simulink model "controled_robot"  (R2018a)
settings: Solver=FixedStepAuto  StartTime=0.0  StopTime=20  FixedStep=0.0001  MaxStep=5e-3  RelTol=1e-3
undefined symbols (not defined in the file or in its folder): DiscIntNeverNeededParam, Forward_Dynamics
libraries: simulink x2
settings Model: Creator=julien  LastModifiedBy=quentin
settings SolverCC: AutoInsertRateTranBlk=on
settings DataIOCC: ReturnWorkspaceOutputs=on  ReturnWorkspaceOutputsName=tpe1c572a4_15fe_4767_8dc5_e730d6ee611a  LoggingIntervals=[10, 20]
settings CodeAppCC: StateflowObjectComments=on

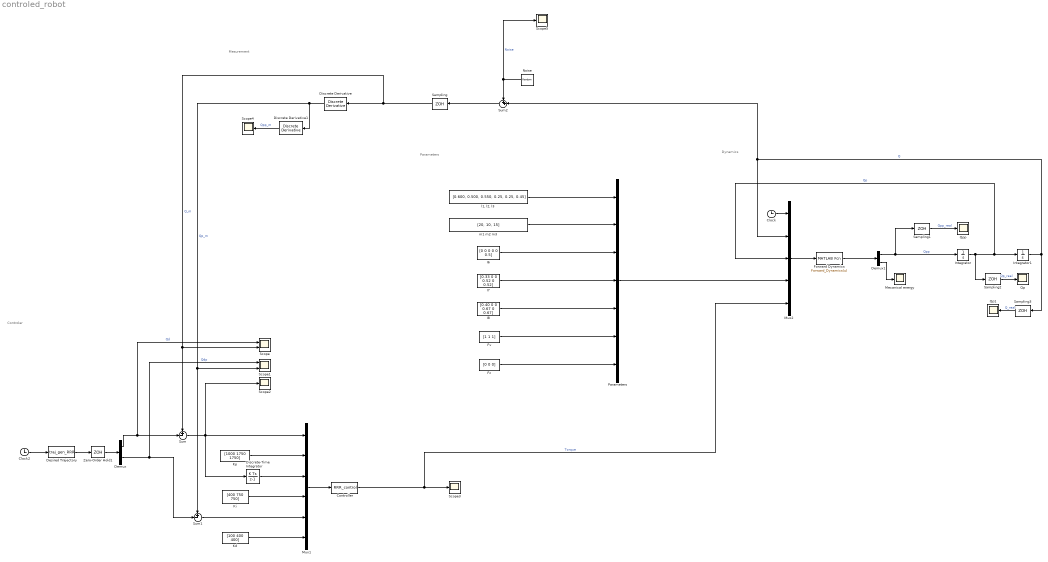
== system controled_robot ==
  note: Parameters
  note: Dynamics
  note: Controler
  note: Mesurement
  Clock : Clock
  Clock2 : Clock
  "Controller " : MATLABFcn  MATLABFcn=RRR_control
  Demux : Demux  Outputs=[3 3]
  Demux1 : Demux  Outputs=[3, 3]
  Desired Trajectory : MATLABFcn  MATLABFcn=traj_gen_RRR  OutputDimensions=6
  Discrete Derivative : simulink/Discrete/Discrete Derivative  gainval=1  ICPrevScaledInput=0.0  OutMin=[]  OutMax=[]  OutDataType=fixdt(1, 16)  OutScaling=2^-10  DoSatur=off
  Discrete Derivative1 : simulink/Discrete/Discrete Derivative  gainval=1  ICPrevScaledInput=0.0  OutMin=[]  OutMax=[]  OutDataType=fixdt(1, 16)  OutScaling=2^-10  DoSatur=off
  Discrete-Time Integrator : DiscreteIntegrator  SampleTime=0.001  ICPrevOutput=DiscIntNeverNeededParam  ICPrevScaledInput=DiscIntNeverNeededParam
  Fc : Constant  Value=[0 0 0]
  Forward Dynamics : MATLABFcn  MATLABFcn=Forward_Dynamics(u)  OutputDimensions=6
  Fv : Constant  Value=[1 1 1]
  I6 : Constant  Value=[0 0 0 0 0 0.5]
  I7 : Constant  Value=[0.33 0 0 0.52 0 0.52]
  I8 : Constant  Value=[0.40 0 0 0.67 0 0.67]
  Integrator : Integrator  InitialCondition=[0,0,0]
  Integrator1 : Integrator  InitialCondition=[0, pi/2, 0.1]
  Kd : Constant  Value=[100 400 400]
  Ki : Constant  Value=[400 750 750]
  Kp : Constant  Value=[1000 1750 1750]
  Mecanical energy : Scope
  Mux1 : Mux  Inputs=6
  Mux2 : Mux  Inputs=5
  Noise : RandomNumber  Mean=[0 0 0]  Variance=1e-3*pi/180*1e-3*pi/180 * [1 1 1]  Seed=[1 2 3]  SampleTime=0.001  VectorParams1D=off
  Parameters : Mux  Inputs=7
  Qp : Scope
  Qp1 : Scope
  Qpp : Scope
  Sampling{,1..3} (4 alike) : ZeroOrderHold  SampleTime=0.001
  Scope : Scope  NumInputPorts=2
  Scope1 : Scope  NumInputPorts=2
  Scope{2..5} (4 alike) : Scope
  Sum : Sum  Inputs=+-|
  Sum1 : Sum  Inputs=+-|
  Sum2 : Sum  Inputs=++|
  Zero-Order Hold1 : ZeroOrderHold  SampleTime=0.001
  "l1, l2, l3" : Constant  Value=[0.600, 0.500, 0.550, 0.25, 0.25, 0.45]
  m1 m2 m3 : Constant  Value=[20, 10, 15]
  wires:
  Clock/1 -> Mux2/1
  Mux2/1 -> Forward Dynamics/1
  Integrator/1 -> Sampling2/1, Mux2/3, Integrator1/1  "Qp"
  Integrator1/1 -> Sampling3/1, Sum2/2, Mux2/2  "Q"
  Clock2/1 -> Desired Trajectory/1
  Desired Trajectory/1 -> Zero-Order Hold1/1
  Demux/1 -> Scope/1, Sum/2  "Qd"
  Demux/2 -> Scope1/1, Sum1/2  "Qdp"
  Sum/1 -> Discrete-Time Integrator/1, Scope2/1, Mux1/1
  Mux1/1 -> "Controller "/1
  Discrete-Time Integrator/1 -> Mux1/3
  Sum1/1 -> Mux1/5
  Kp/1 -> Mux1/2
  Ki/1 -> Mux1/4
  Kd/1 -> Mux1/6
  Forward Dynamics/1 -> Demux1/1
  Demux1/1 -> Sampling1/1, Integrator/1  "Qpp"
  Demux1/2 -> Mecanical energy/1
  "l1, l2, l3"/1 -> Parameters/1
  m1 m2 m3/1 -> Parameters/2
  I6/1 -> Parameters/3
  I7/1 -> Parameters/4
  I8/1 -> Parameters/5
  Fv/1 -> Parameters/6
  Fc/1 -> Parameters/7
  "Controller "/1 -> Scope3/1, Mux2/5  "Torque"
  Parameters/1 -> Mux2/4
  Sampling/1 -> Scope/2, Sum/1, Discrete Derivative/1  "Q_m"
  Discrete Derivative/1 -> Discrete Derivative1/1, Sum1/1, Scope1/2  "Qp_m"
  Zero-Order Hold1/1 -> Demux/1
  Sum2/1 -> Sampling/1
  Noise/1 -> Scope5/1, Sum2/1  "Noise"
  Discrete Derivative1/1 -> Scope4/1  "Qpp_m"
  Sampling1/1 -> Qpp/1  "Qpp_real"
  Sampling2/1 -> Qp/1  "Qp_real"
  Sampling3/1 -> Qp1/1  "Q_real"
